simulink model "Fuzz_PID_Sys"  (R2021a)
settings: Solver=VariableStepAuto  StartTime=0.0  StopTime=200  RelTol=1e-3
undefined symbols (not defined in the file or in its folder): DiscIntNeverNeededParam
libraries: fuzblock x7, simulink x2
settings Model: Creator=Le_旭  LastModifiedBy=WU
settings SolverCC: AlgebraicLoopSolver=TrustRegion
settings DebuggingCC: SFMachineParentedDataDiag=warning

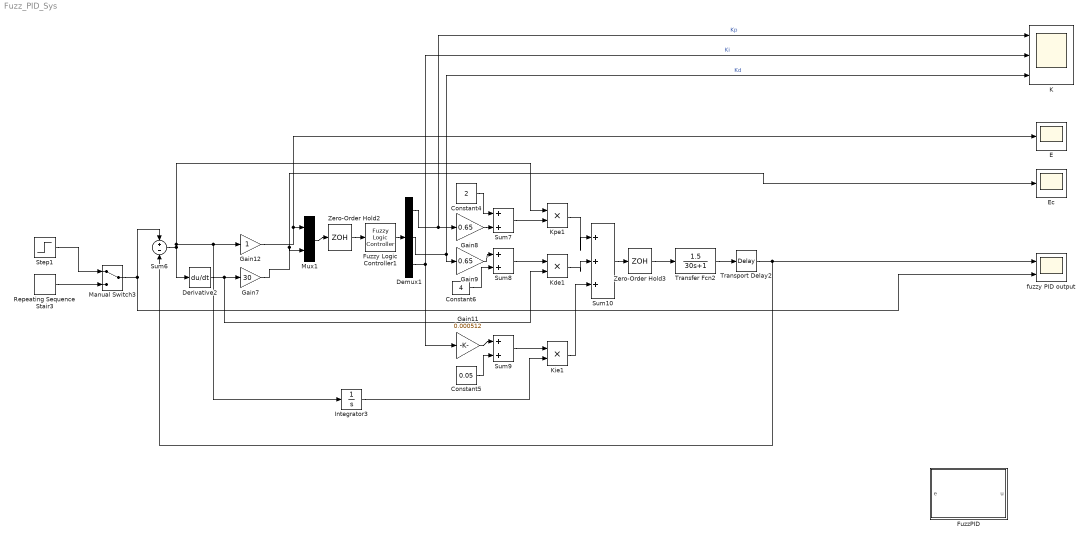
== system Fuzz_PID_Sys ==
  Constant4 : Constant  Value=2
  Constant5 : Constant  Value=0.05
  Constant6 : Constant  Value=4
  Demux1 : Demux  Outputs=3
      settings: DisplayOption=none
  Derivative2 : Derivative
  E : Scope
  Ec : Scope
  FuzzPID : Subsystem
  Fuzzy Logic Controller1 : fuzblock/Fuzzy Logic  Controller  FIS='fuzzyPID'  OutputSampleNumber=101  DataType=double  FuzzifiedInputs=off  RuleFiringStrengths=off  RuleOutputs=off  AggregatedOutputs=off  SimulateUsing=Interpreted execution  OutOfRangeInputValueMessage=warning  NoRuleFiredMessage=warning  EmptyOutputFuzzySetMessage=warning
  Gain11 : Gain  Gain=0.000512  SaturateOnIntegerOverflow=on  OutDataTypeStr=Inherit: Same as input  ParamDataTypeStr=Inherit: Same as input
  Gain12 : Gain  SaturateOnIntegerOverflow=on  OutDataTypeStr=Inherit: Same as input  ParamDataTypeStr=Inherit: Same as input
  Gain7 : Gain  Gain=30  SaturateOnIntegerOverflow=on  OutDataTypeStr=Inherit: Same as input  ParamDataTypeStr=Inherit: Same as input
  Gain8 : Gain  Gain=0.65  SaturateOnIntegerOverflow=on  OutDataTypeStr=Inherit: Same as input  ParamDataTypeStr=Inherit: Same as input
  Gain9 : Gain  Gain=0.65  SaturateOnIntegerOverflow=on  OutDataTypeStr=Inherit: Same as input  ParamDataTypeStr=Inherit: Same as input
  Integrator3 : Integrator
  K : Scope  NumInputPorts=3
  Kde1 : Product  SaturateOnIntegerOverflow=on  OutDataTypeStr=Inherit: Same as first input
  Kie1 : Product  SaturateOnIntegerOverflow=on  OutDataTypeStr=Inherit: Same as first input
  Kpe1 : Product  SaturateOnIntegerOverflow=on  OutDataTypeStr=Inherit: Same as first input
  Manual Switch3 : ManualSwitch
  Mux1 : Mux  Inputs=2
  Repeating Sequence Stair3 : simulink/Sources/Repeating Sequence Stair  OutValues=[8 1 1 2 2 ].'  tsamp=20  OutMin=[]  OutMax=[]  OutDataTypeStr=double  OutputDataTypeScalingMode=double  OutDataType=fixdt(0,8)  ConRadixGroup=Best Precision: Vector-wise  OutScaling=2^-12
  Step1 : Step  Time=0  SampleTime=0
  Sum10 : Sum  Inputs=|+++  SaturateOnIntegerOverflow=on
  Sum6 : Sum  Inputs=+-  SaturateOnIntegerOverflow=on
  Sum7 : Sum  Inputs=|++  SaturateOnIntegerOverflow=on
  Sum8 : Sum  Inputs=|++  SaturateOnIntegerOverflow=on
  Sum9 : Sum  Inputs=|++  SaturateOnIntegerOverflow=on
  Transfer Fcn2 : TransferFcn  Numerator=[1.5]  Denominator=[30 1]
  Transport Delay2 : TransportDelay  DelayTime=10  BufferSize=1000000
  Zero-Order Hold2 : ZeroOrderHold  SampleTime=0.1
  Zero-Order Hold3 : ZeroOrderHold  SampleTime=0.1
  fuzzy PID output : Scope  NumInputPorts=2
  wires:
  Gain12/1 -> Mux1/1, E/1
  Demux1/1 -> K/1, Gain8/1  "Kp"
  Mux1/1 -> Zero-Order Hold2/1
  Gain7/1 -> Ec/1, Mux1/2
  Demux1/3 -> K/2, Gain11/1  "Ki"
  Zero-Order Hold2/1 -> Fuzzy Logic Controller1/1
  Sum6/1 -> Kpe1/1, Integrator3/1, Gain12/1, Derivative2/1
  Sum9/1 -> Kie1/1
  Gain8/1 -> Sum7/2
  Kde1/1 -> Sum10/2
  Demux1/2 -> K/3, Gain9/1  "Kd"
  Kie1/1 -> Sum10/3
  Transport Delay2/1 -> Sum6/2, fuzzy PID output/1
  Kpe1/1 -> Sum10/1
  Sum10/1 -> Zero-Order Hold3/1
  Gain9/1 -> Sum8/1
  Constant6/1 -> Sum8/2
  Integrator3/1 -> Kie1/2
  Gain11/1 -> Sum9/1
  Constant4/1 -> Sum7/1
  Fuzzy Logic Controller1/1 -> Demux1/1
  Constant5/1 -> Sum9/2
  Step1/1 -> Manual Switch3/1
  Sum7/1 -> Kpe1/2
  Sum8/1 -> Kde1/1
  Derivative2/1 -> Kde1/2, Gain7/1
  Repeating Sequence Stair3/1 -> Manual Switch3/2
  Manual Switch3/1 -> Sum6/1, fuzzy PID output/2
  Zero-Order Hold3/1 -> Transfer Fcn2/1
  Transfer Fcn2/1 -> Transport Delay2/1

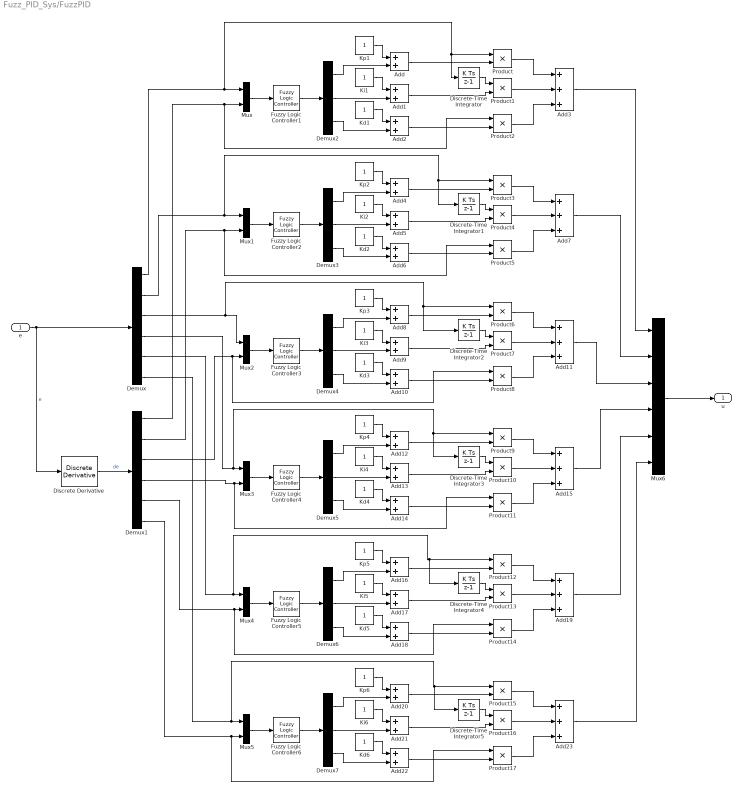
== system Fuzz_PID_Sys/FuzzPID ==
  e : Inport
  Add{,1..2,4..6,8..10,12..14,16..18,20..22} (18 alike) : Sum
  Add{3,7,11,15,19,23} (6 alike) : Sum  Inputs=+++
  Demux : Demux  Outputs=6
      settings: DisplayOption=none
  Demux1 : Demux  Outputs=6
      settings: DisplayOption=none
  Demux{2..7} (6 alike) : Demux  Outputs=3
      settings: DisplayOption=none
  Discrete Derivative : simulink/Discrete/Discrete Derivative  gainval=1.0  ICPrevScaledInput=0.0  OutMin=[]  OutMax=[]  OutDataType=fixdt(1, 16)  OutScaling=2^-10  DoSatur=off
  Discrete-Time Integrator{,1..5} (6 alike) : DiscreteIntegrator  SampleTime=-1  ICPrevOutput=DiscIntNeverNeededParam  ICPrevScaledInput=DiscIntNeverNeededParam
  Fuzzy Logic Controller{1..6} (6 alike) : fuzblock/Fuzzy Logic  Controller  FIS='fuzzyPID'  OutputSampleNumber=101  DataType=double  FuzzifiedInputs=off  RuleFiringStrengths=off  RuleOutputs=off  AggregatedOutputs=off  SimulateUsing=Interpreted execution  OutOfRangeInputValueMessage=warning  NoRuleFiredMessage=warning  EmptyOutputFuzzySetMessage=warning
  Kd{1..6} (6 alike) : Constant
  Ki{1..6} (6 alike) : Constant
  Kp{1..6} (6 alike) : Constant
  Mux{,1..5} (6 alike) : Mux  Inputs=2
  Mux6 : Mux  Inputs=6
  Product{,1..17} (18 alike) : Product
  u : Outport
  wires:
  e/1 -> Discrete Derivative/1, Demux/1  "e"
  Discrete Derivative/1 -> Demux1/1  "de"
  Mux/1 -> Fuzzy Logic Controller1/1
  Fuzzy Logic Controller1/1 -> Demux2/1
  Demux2/1 -> Add/2
  Kp1/1 -> Add/1
  Ki1/1 -> Add1/1
  Demux2/2 -> Add1/2
  Kd1/1 -> Add2/1
  Demux2/3 -> Add2/2
  Add/1 -> Product/2
  Discrete-Time Integrator/1 -> Product1/1
  Add1/1 -> Product1/2
  Add2/1 -> Product2/2
  Product1/1 -> Add3/2
  Product/1 -> Add3/1
  Product2/1 -> Add3/3
  Product5/1 -> Add7/3
  Product4/1 -> Add7/2
  Product3/1 -> Add7/1
  Kd2/1 -> Add6/1
  Kp2/1 -> Add4/1
  Discrete-Time Integrator1/1 -> Product4/1
  Add4/1 -> Product3/2
  Demux3/3 -> Add6/2
  Fuzzy Logic Controller2/1 -> Demux3/1
  Demux3/1 -> Add4/2
  Add5/1 -> Product4/2
  Add6/1 -> Product5/2
  Mux1/1 -> Fuzzy Logic Controller2/1
  Demux3/2 -> Add5/2
  Ki2/1 -> Add5/1
  Product8/1 -> Add11/3
  Product7/1 -> Add11/2
  Product6/1 -> Add11/1
  Kd3/1 -> Add10/1
  Kp3/1 -> Add8/1
  Discrete-Time Integrator2/1 -> Product7/1
  Add8/1 -> Product6/2
  Demux4/3 -> Add10/2
  Fuzzy Logic Controller3/1 -> Demux4/1
  Demux4/1 -> Add8/2
  Add9/1 -> Product7/2
  Add10/1 -> Product8/2
  Mux2/1 -> Fuzzy Logic Controller3/1
  Demux4/2 -> Add9/2
  Ki3/1 -> Add9/1
  Product11/1 -> Add15/3
  Product10/1 -> Add15/2
  Product9/1 -> Add15/1
  Kd4/1 -> Add14/1
  Kp4/1 -> Add12/1
  Discrete-Time Integrator3/1 -> Product10/1
  Add12/1 -> Product9/2
  Demux5/3 -> Add14/2
  Fuzzy Logic Controller4/1 -> Demux5/1
  Demux5/1 -> Add12/2
  Add13/1 -> Product10/2
  Add14/1 -> Product11/2
  Mux3/1 -> Fuzzy Logic Controller4/1
  Demux5/2 -> Add13/2
  Ki4/1 -> Add13/1
  Product14/1 -> Add19/3
  Product13/1 -> Add19/2
  Product12/1 -> Add19/1
  Kd5/1 -> Add18/1
  Kp5/1 -> Add16/1
  Discrete-Time Integrator4/1 -> Product13/1
  Add16/1 -> Product12/2
  Demux6/3 -> Add18/2
  Fuzzy Logic Controller5/1 -> Demux6/1
  Demux6/1 -> Add16/2
  Add17/1 -> Product13/2
  Add18/1 -> Product14/2
  Mux4/1 -> Fuzzy Logic Controller5/1
  Demux6/2 -> Add17/2
  Ki5/1 -> Add17/1
  Product17/1 -> Add23/3
  Product16/1 -> Add23/2
  Product15/1 -> Add23/1
  Kd6/1 -> Add22/1
  Kp6/1 -> Add20/1
  Discrete-Time Integrator5/1 -> Product16/1
  Add20/1 -> Product15/2
  Demux7/3 -> Add22/2
  Fuzzy Logic Controller6/1 -> Demux7/1
  Demux7/1 -> Add20/2
  Add21/1 -> Product16/2
  Add22/1 -> Product17/2
  Mux5/1 -> Fuzzy Logic Controller6/1
  Demux7/2 -> Add21/2
  Ki6/1 -> Add21/1
  Demux/1 -> Discrete-Time Integrator/1, Product/1, Mux/1
  Demux/2 -> Discrete-Time Integrator1/1, Product3/1, Mux1/1
  Demux/3 -> Discrete-Time Integrator2/1, Product6/1, Mux2/1
  Demux/4 -> Discrete-Time Integrator3/1, Product9/1, Mux3/1
  Demux/5 -> Discrete-Time Integrator4/1, Product12/1, Mux4/1
  Demux/6 -> Discrete-Time Integrator5/1, Product15/1, Mux5/1
  Demux1/1 -> Product2/1, Mux/2
  Demux1/2 -> Product5/1, Mux1/2
  Demux1/3 -> Product8/1, Mux2/2
  Demux1/4 -> Product11/1, Mux3/2
  Demux1/5 -> Product14/1, Mux4/2
  Demux1/6 -> Product17/1, Mux5/2
  Add3/1 -> Mux6/1
  Add7/1 -> Mux6/2
  Add11/1 -> Mux6/3
  Add15/1 -> Mux6/4
  Add19/1 -> Mux6/5
  Add23/1 -> Mux6/6
  Mux6/1 -> u/1
